simulink model "sl_chart"  (Simulink 6.6)
settings: Solver=FixedStepDiscrete  StartTime=0.0  StopTime=10.0  RelTol=1e-3
settings Model: Creator=volgy  LastModifiedBy=vBuskirk
settings DebuggingCC: MultiTaskCondExecSysMsg=none
settings RTWCC: IncludeERTFirstTime=on

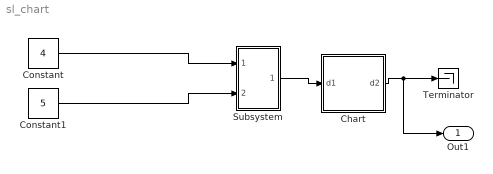
== system sl_chart ==
  Chart : Stateflow chart
  Constant : Constant  Value=4
  Constant1 : Constant  Value=5
  Subsystem : Subsystem
  Terminator : Terminator
  Out1 : Outport
  wires:
  Constant/1 -> Subsystem/1(In1)
  Constant1/1 -> Subsystem/2(In2)
  Subsystem/1(Out1) -> Chart/1(d1)
  Chart/1(d2) -> Out1/1, Terminator/1

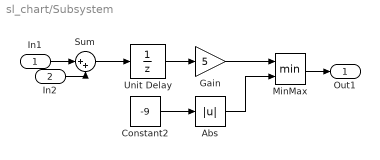
== system sl_chart/Subsystem ==
  In1 : Inport
  In2 : Inport  Port=2
  Abs : Abs
  Constant2 : Constant  Value=-9
  Gain : Gain  Gain=5
  MinMax : MinMax  Inputs=2
  Sum : Sum  Inputs=|++
  Unit Delay : UnitDelay
  Out1 : Outport
  wires:
  Constant2/1 -> Abs/1
  Gain/1 -> MinMax/1
  Abs/1 -> MinMax/2
  Sum/1 -> Unit Delay/1
  Unit Delay/1 -> Gain/1
  In1/1 -> Sum/1
  MinMax/1 -> Out1/1
  In2/1 -> Sum/2

== stateflow chart Chart ==
  state s1
  state s2
  (default) -> s1
  s1 -> s2 : [d1 == 5]/ d2 = 8
  data: d1 input inherited; d2 output double
